simulink model "LateralControllerCheck"  (R2018a)
settings: Solver=ode4  StartTime=0.0  StopTime=500  FixedStep=0.001  RelTol=1e-3
values from neighbouring files (symbols this model uses):
  g = aircraft_data(52)    [TF.m]    (also in param_code.m)
  U0 = s0(1)    [TF.m]    (also in param_code.m)
libraries: simulink_extras x4, cstblocks x3
settings Model: Creator=engmh  LastModifiedBy=engmh
settings DataIOCC: ReturnWorkspaceOutputs=on
settings DebuggingCC: SFMachineParentedDataDiag=error
settings SFSimCC: SimUseLocalCustomCode=on
settings RTWCC: RTWUseLocalCustomCode=on

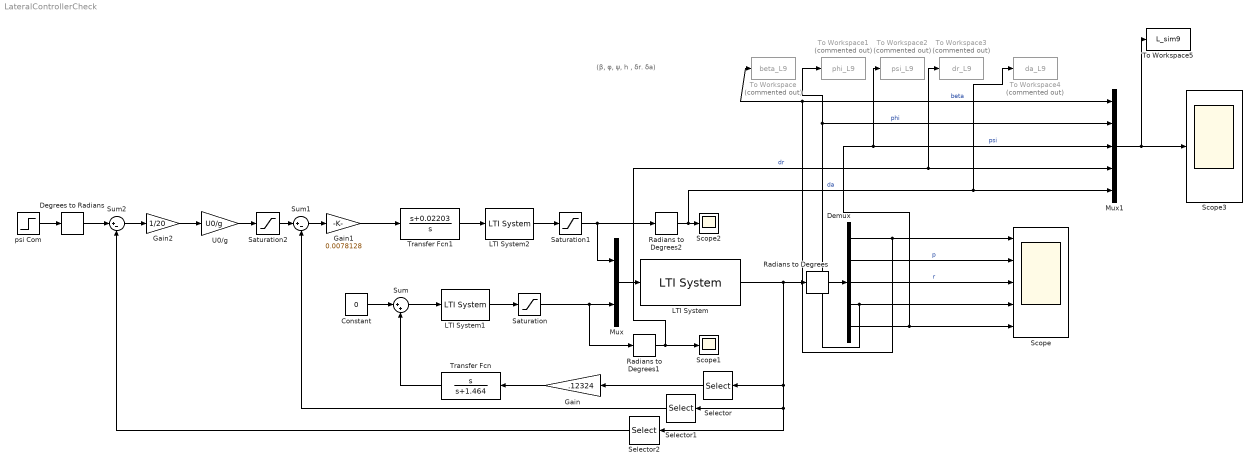
== system LateralControllerCheck ==
  note: (β, φ, ψ, h , δr. δa)
  Constant : Constant  Value=0
  Degrees to Radians : simulink_extras/Transformations/Degrees to Radians
  Demux : Demux  Outputs=5
  Gain : Gain  Gain=.12324
  Gain1 : Gain  Gain=0.0078128
  Gain2 : Gain  Gain=1/20
  LTI System : cstblocks/LTI System  sys=Lateral_SS  IC=[]
  LTI System1 : cstblocks/LTI System  sys=servo  IC=[]
  LTI System2 : cstblocks/LTI System  sys=servo  IC=[]
  Mux : Mux  Inputs=2
  Mux1 : Mux  Inputs=5
  Radians to Degrees : simulink_extras/Transformations/Radians to Degrees
  Radians to Degrees1 : simulink_extras/Transformations/Radians to Degrees
  Radians to Degrees2 : simulink_extras/Transformations/Radians to Degrees
  Saturation : Saturate  UpperLimit=15*pi/180  LowerLimit=-15*pi/180
  Saturation1 : Saturate  UpperLimit=50*pi/180  LowerLimit=-50*pi/180
  Saturation2 : Saturate  UpperLimit=30*pi/180  LowerLimit=-30*pi/180
  Scope : Scope  NumInputPorts=5
  Scope1 : Scope
  Scope2 : Scope
  Scope3 : Scope
  Selector : Selector  InputPortWidth=5  IndexOptions=Index vector (dialog)  Indices=[3]  OutputSizes=1
  Selector1 : Selector  InputPortWidth=5  IndexOptions=Index vector (dialog)  Indices=[4]  OutputSizes=1
  Selector2 : Selector  InputPortWidth=5  IndexOptions=Index vector (dialog)  Indices=[5]  OutputSizes=1
  Sum : Sum  Inputs=|++
  Sum1 : Sum  Inputs=|+-
  Sum2 : Sum  Inputs=|+-
  To Workspace : ToWorkspace  Commented=on  VariableName=beta_L9  SampleTime=-1
      settings: Save2DSignal=2-D array (concatenate along first dimension)
  To Workspace1 : ToWorkspace  Commented=on  VariableName=phi_L9  SampleTime=-1
      settings: Save2DSignal=2-D array (concatenate along first dimension)
  To Workspace2 : ToWorkspace  Commented=on  VariableName=psi_L9  SampleTime=-1
      settings: Save2DSignal=2-D array (concatenate along first dimension)
  To Workspace3 : ToWorkspace  Commented=on  VariableName=dr_L9  SampleTime=-1
      settings: Save2DSignal=2-D array (concatenate along first dimension)
  To Workspace4 : ToWorkspace  Commented=on  VariableName=da_L9  SampleTime=-1
      settings: Save2DSignal=2-D array (concatenate along first dimension)
  To Workspace5 : ToWorkspace  VariableName=L_sim9  SaveFormat=Timeseries  SampleTime=-1
      settings: Save2DSignal=2-D array (concatenate along first dimension)
  Transfer Fcn : TransferFcn  Numerator=[1 0]  Denominator=[1 1.464]
  Transfer Fcn1 : TransferFcn  Numerator=[1 0.02203]  Denominator=[1 0]
  U0/g : Gain  Gain=U0/g
  "psi Com " : Step  Time=0  After=360  SampleTime=0
  wires:
  Gain/1 -> Transfer Fcn/1
  LTI System/1 -> Selector2/1, Selector1/1, Selector/1, Radians to Degrees/1
  Selector/1 -> Gain/1
  Transfer Fcn/1 -> Sum/2
  Constant/1 -> Sum/1
  Sum/1 -> LTI System1/1
  LTI System1/1 -> Saturation/1
  Mux/1 -> LTI System/1
  Saturation/1 -> Radians to Degrees1/1, Mux/2
  Demux/1 -> Mux1/1, To Workspace/1, Scope/1  "beta"
  Demux/2 -> Scope/2  "p"
  Demux/3 -> Scope/3  "r"
  Demux/4 -> Scope/4, Mux1/2, To Workspace1/1  "phi"
  Demux/5 -> Mux1/3, To Workspace2/1, Scope/5  "psi"
  LTI System2/1 -> Saturation1/1
  Selector1/1 -> Sum1/2
  Saturation1/1 -> Radians to Degrees2/1, Mux/1
  Gain1/1 -> Transfer Fcn1/1
  Sum1/1 -> Gain1/1
  Transfer Fcn1/1 -> LTI System2/1
  Sum2/1 -> Gain2/1
  Gain2/1 -> U0/g/1
  Selector2/1 -> Sum2/2
  "psi Com "/1 -> Degrees to Radians/1
  Degrees to Radians/1 -> Sum2/1
  Radians to Degrees/1 -> Demux/1
  Radians to Degrees1/1 -> Mux1/4, To Workspace3/1, Scope1/1  "dr"
  U0/g/1 -> Saturation2/1
  Saturation2/1 -> Sum1/1
  Radians to Degrees2/1 -> Mux1/5, To Workspace4/1, Scope2/1  "da"
  Mux1/1 -> To Workspace5/1, Scope3/1
